simulink model "F4_DAC_WriteDma"  (R2018b)
settings: Solver=FixedStepDiscrete  StartTime=0.0  StopTime=10.0  RelTol=1e-3  EnableMultiTasking=on
libraries: DAC_Lib x1, STM32_Config_Lib x1, TIMERS_Lib x1
settings Model: Creator=reynaudp  LastModifiedBy=fenard1
settings DataIOCC: LimitDataPoints=on
settings OptimizationCC: DefaultParameterBehavior=Inlined  DefaultUnderspecifiedDataType=single  PassReuseOutputArgsAs=Individual arguments  LifeSpan=1
settings DebuggingCC: UniqueDataStoreMsg=error  AllowSymbolicDim=off  StrictBusMsg=ErrorOnBusTreatedAsVector  SFUnexpectedBacktrackingDiag=warning  SFNoUnconditionalDefaultTransitionDiag=warning  SFUndirectedBroadcastEventsDiag=error  SFExecutionAtInitializationDiag=none
settings HardwareCC: ProdBitPerPointer=32  ProdBitPerSizeT=32  ProdBitPerPtrDiffT=32  ProdLargestAtomicInteger=Integer  ProdWordSize=32  ProdHWDeviceType=STMicroelectronics->STM32 32-bit Cortex-M
settings ModelReferenceCC: PropagateSignalLabelsOutOfModel=off
settings SFSimCC: SimUseLocalCustomCode=off  CompileTimeRecursionLimit=0  EnableRuntimeRecursion=off  MATLABDynamicMemAlloc=off
settings RTWCC: SystemTargetFile=stm32.tlc  TemplateMakefile=stm32.tmf  Description=stm32 (Embedded Target)  GenerateReport=on  RTWUseLocalCustomCode=off
settings CodeAppCC: IgnoreCustomStorageClasses=off  CustomSymbolStrType=$N$R$M  ParamNamingRule=UpperCase  SimulinkBlockComments=off
settings STFCustomTargetCC: TargetLangStandard=C99 (ISO)  ParMdlRefBuildCompliant=on  IncludeMdlTerminateFcn=off  CombineOutputUpdateFcns=on  ERTCustomFileBanners=on  SupportContinuousTime=off  SupportNonInlinedSFcns=off  RemoveResetFunc=on  ParenthesesLevel=Maximum  CastingMode=Standards  MATLABClassNameForMDSCustomization=Simulink.SoftwareTarget.ERTCustomization  SystemTargetFile=stm32.tlc
settings ERTTargetCC: TargetLangStandard=C99 (ISO)  MultiwordLength=2048  CompOptLevelCompliant=off  ConcurrentExecutionCompliant=off  IncludeMdlTerminateFcn=off  ParenthesesLevel=Maximum  CastingMode=Standards  ModelStepFunctionPrototypeControlCompliant=off  CPPClassGenCompliant=off  UseToolchainInfoCompliant=off  InlinedParameterPlacement=NonHierarchical  ERTSrcFileBannerTemplate=sourceFileTemplate.cgt  ERTHdrFileBannerTemplate=sourceFileTemplate.cgt  ERTDataSrcFileTemplate=sourceFileTemplate.cgt  ERTDataHdrFileTemplate=sourceFileTemplate.cgt  ERTCustomFileTemplate=customRoutineProcess.tlc  ConvertIfToSwitch=off  SuppressUnreachableDefaultCases=off  EnableSignedLeftShifts=off  EnableSignedRightShifts=off
settings ConfigComp: CovMetricSettings=dw  CovHtmlReporting=on  CovSaveCumulativeToWorkspaceVar=on  CovSaveSingleToWorkspaceVar=on  CovExternalEMLEnable=off

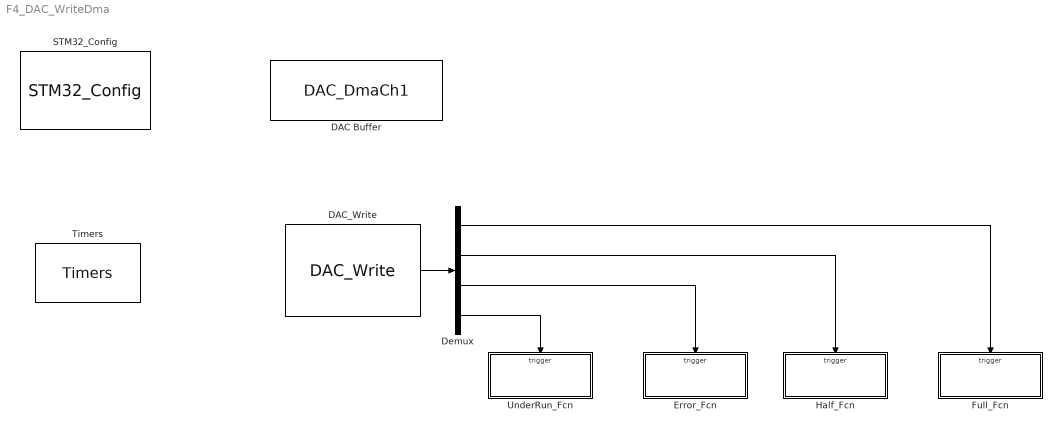
== system F4_DAC_WriteDma ==
  DAC Buffer : DataStoreMemory  Priority=1  DataStoreName=DAC_DmaCh1  ReadBeforeWriteMsg=warning  WriteAfterWriteMsg=warning  WriteAfterReadMsg=warning  InitialValue=[10 20 30 40 50 60 70 80 90 100 ]  ShowAdditionalParam=off  OutDataTypeStr=uint16
      settings: AttributesFormatString=Priority=%<Priority>  RTWStateStorageClass=ImportedExternPointer
  DAC_Write : DAC_Lib/DAC_Write  Priority=2  DAC_Name=DAC  Pin0=off  Pin1=off  Align=12bit_right  DmaBuffCh1=10  DmaBuffCh2=0  CpltTrans=on  HalfTrans=on  ErrorIt=on  UnderIt=on  NbDAC=1  UsedDma=on
      settings: AttributesFormatString=Priority=%<Priority>  SourceProductName=Target Support Package - STM32 Adapter
  Demux : Demux
  Error_Fcn : Subsystem  TreatAsAtomicUnit=on
  "Full_Fcn " : Subsystem  TreatAsAtomicUnit=on
  Half_Fcn : Subsystem  TreatAsAtomicUnit=on
  STM32_Config : STM32_Config_Lib/STM32_Config  Priority=0  Project_Path=.\  Config_File=F4_DAC_WriteDma.ioc  MCU_Name=STM32F407VGTx
      settings: SourceProductName=Target Support Package - STM32 Adapter
  Timers : TIMERS_Lib/Timers  Priority=3  currentTIM=TIM2  TIM_Name=TIM2  sysUsingTimer=on  TIM_APBClock=84000000  TIM_Set_Clk=off  TIM_Prescaler=84-1  TIM_Clock=1000000.00  Variable_frequency=off  TIM_Set_OutFreq=off  TIM_ARR=1000  Output_frequency=1000.00  Repetition_counter=0  TIM_Mode=Up  TIM_DMA=none  TIM_IRQ=off  TIM_IRQ_ONLY=on  TIM_UP=off  TIM_TRG=off  TIM_COM=off  TIM_BRK=off  NbTIM=1  CH1_enable=off  CH1N_enable=off  CH1_type=Unknown  CH1_DMA=off  CH1_int=off  CH1_edge=Rising  CH1_div=1  CH1_variable_duty=off  CH1_set_pulse=off  CH1_output_duty=0.00  CH1_pulse=0  CH2_enable=off  CH2N_enable=off  CH2_type=Unknown  CH2_DMA=off  CH2_int=off  CH2_edge=Rising  CH2_div=1  CH2_variable_duty=off  CH2_set_pulse=off  CH2_output_duty=0.00  CH2_pulse=0  CH3_enable=off  CH3N_enable=off  CH3_type=Unknown  CH3_DMA=off  CH3_int=off  CH3_edge=Rising  CH3_div=1  CH3_variable_duty=off  CH3_set_pulse=off  CH3_output_duty=0.00  CH3_pulse=0  CH4_enable=off  CH4N_enable=off  CH4_type=Unknown  CH4_DMA=off  CH4_int=off  CH4_edge=Rising  CH4_div=1  CH4_variable_duty=off  CH4_set_pulse=off  CH4_output_duty=0.00  CH4_pulse=0
      settings: AttributesFormatString=Priority=%<Priority>  SourceProductName=Target Support Package - STM32 Adapter
  UnderRun_Fcn : Subsystem  TreatAsAtomicUnit=on
  wires:
  Demux/3 -> Error_Fcn/Trigger
  Demux/2 -> Half_Fcn/Trigger
  Demux/4 -> UnderRun_Fcn/Trigger
  DAC_Write/1 -> Demux/1
  Demux/1 -> "Full_Fcn "/Trigger

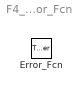
== system F4_DAC_WriteDma/Error_Fcn ==
  Error_Fcn : TriggerPort  TriggerType=function-call  VariantControl=Variant

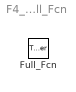
== system F4_DAC_WriteDma/Full_Fcn  ==
  Full_Fcn : TriggerPort  TriggerType=function-call  VariantControl=Variant

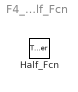
== system F4_DAC_WriteDma/Half_Fcn ==
  Half_Fcn : TriggerPort  TriggerType=function-call  VariantControl=Variant

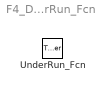
== system F4_DAC_WriteDma/UnderRun_Fcn ==
  UnderRun_Fcn : TriggerPort  TriggerType=function-call  VariantControl=Variant
